simulink model "fast_test"  (R2022a)
settings: Solver=VariableStepAuto  StartTime=0.0  StopTime=25  RelTol=1e-3
undefined symbols (not defined in the file or in its folder): W_driver
libraries: cstblocks x6, RCTblocks x2
settings Model: Creator=Jonas  LastModifiedBy=Jonas

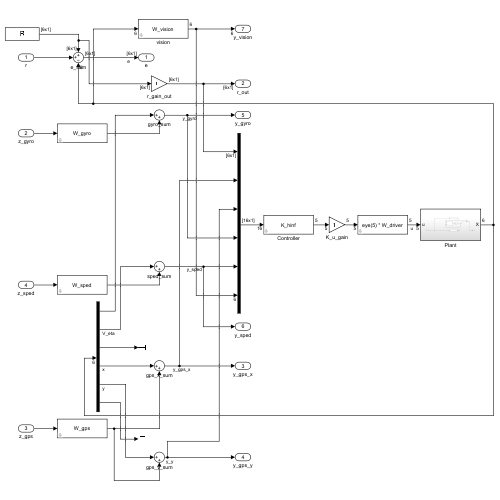
[thumbnail: Simulink's stored preview of the top-level diagram]
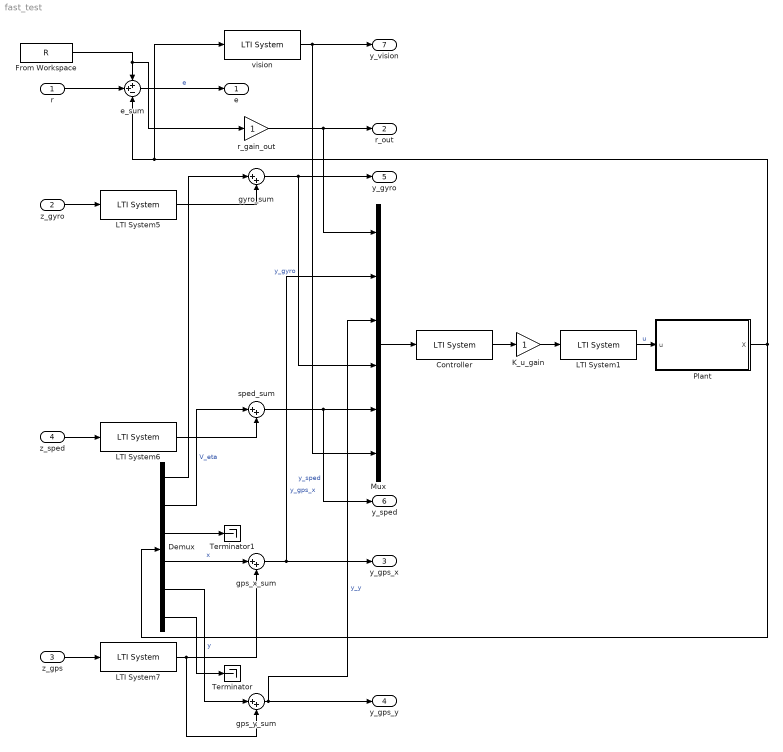
== system fast_test ==
  r : Inport
  z_gyro : Inport  Port=2
  z_gps : Inport  Port=3
  z_sped : Inport  Port=4
  Controller : cstblocks/LTI System  sys=K_hinf  IC=[]
  Demux : Demux  Outputs=6
  From Workspace : FromWorkspace  VariableName=R
  K_u_gain : Gain
  LTI System1 : cstblocks/LTI System  sys=eye(5) * W_driver  IC=[]
  LTI System5 : cstblocks/LTI System  sys=W_gyro  IC=[]
  LTI System6 : cstblocks/LTI System  sys=W_sped  IC=[]
  LTI System7 : cstblocks/LTI System  sys=W_gps  IC=[]
  Mux : Mux  Inputs=6
  Plant : Subsystem
  Terminator : Terminator
  Terminator1 : Terminator
  e_sum : Sum  Inputs=++-
  gps_x_sum : Sum  Inputs=|++
  gps_y_sum : Sum  Inputs=|++
  gyro_sum : Sum  Inputs=|++
  r_gain_out : Gain
  sped_sum : Sum  Inputs=|++
  vision : cstblocks/LTI System  sys=W_vision  IC=[]
  e : Outport
  r_out : Outport  Port=2
  y_gps_x : Outport  Port=3
  y_gps_y : Outport  Port=4
  y_gyro : Outport  Port=5
  y_sped : Outport  Port=6  PortDimensions=1
  y_vision : Outport  Port=7
  wires:
  Mux/1 -> Controller/1
  r/1 -> e_sum/2
  Demux/1 -> gyro_sum/1
  z_sped/1 -> LTI System6/1
  From Workspace/1 -> r_gain_out/1, e_sum/1
  LTI System5/1 -> gyro_sum/2
  z_gps/1 -> LTI System7/1
  Demux/4 -> gps_x_sum/1  "x"
  Demux/5 -> gps_y_sum/1  "y"
  Demux/2 -> sped_sum/1  "V_eta"
  z_gyro/1 -> LTI System5/1
  Demux/3 -> Terminator1/1
  Demux/6 -> Terminator/1
  LTI System6/1 -> sped_sum/2
  Controller/1 -> K_u_gain/1
  r_gain_out/1 -> r_out/1, Mux/1
  LTI System7/1 -> gps_y_sum/2, gps_x_sum/2
  e_sum/1 -> e/1  "e"
  gps_y_sum/1 -> y_gps_y/1, Mux/3  "y_y"
  gyro_sum/1 -> y_gyro/1, Mux/4  "y_gyro"
  sped_sum/1 -> y_sped/1, Mux/5  "y_sped"
  gps_x_sum/1 -> y_gps_x/1, Mux/2  "y_gps_x"
  vision/1 -> y_vision/1, Mux/6
  K_u_gain/1 -> LTI System1/1
  Plant/1(X) -> Demux/1, vision/1, e_sum/3
  LTI System1/1 -> Plant/1(u)  "u"

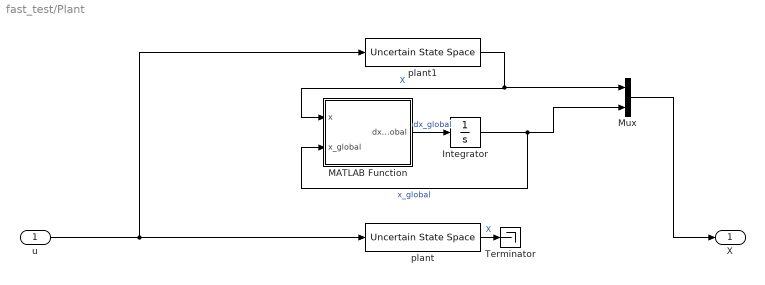
== system fast_test/Plant ==
  u : Inport
  Integrator : Integrator
  MATLAB Function : MATLAB Function  TreatAsAtomicUnit=on
  Mux : Mux  Inputs=2
  Terminator : Terminator
  plant : RCTblocks/Uncertain State Space  Tag=USS  USystem=sys_plant_u  UValue=[]  X0=[]  uX0=[]
      settings: SourceProductBaseCode=RC
  plant1 : RCTblocks/Uncertain State Space  Tag=USS  USystem=sys_plant_u_local  UValue=[]  X0=[]  uX0=[]
      settings: SourceProductBaseCode=RC
  X : Outport
  wires:
  u/1 -> plant1/1, plant/1
  plant1/1 -> Mux/1, MATLAB Function/1(x)  "X"
  MATLAB Function/1(dx_global) -> Integrator/1  "dx_global"
  Integrator/1 -> MATLAB Function/2(x_global), Mux/2  "x_global"
  Mux/1 -> X/1
  plant/1 -> Terminator/1  "X"

== matlab function fast_test/Plant/MATLAB Function ==
  data: x input; dx_global output; x_global input
function dx_global = local2global(x,x_global)
    V_zeta = x(2);
    V_eta = x(3);
    theta = x(4);
    dx_global = x_global;
    dx_global(1) = -V_zeta * cos(theta) + V_eta * sin(theta);
    dx_global(2) = V_eta * cos(theta) + V_zeta * sin(theta);
